simulink model "ExperimentTwoBD"  (R2015a)
settings: Solver=ode45  StartTime=0.0  StopTime=40.0  RelTol=1e-3
settings Model: Creator=Abdullah  LastModifiedBy=Abdullah

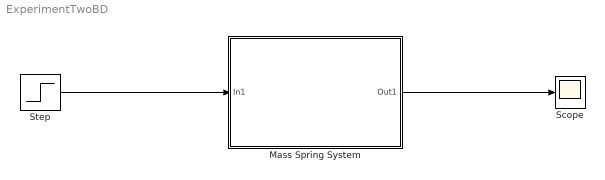
== system ExperimentTwoBD ==
  Mass Spring System : Subsystem
  Scope : Scope
  Step : Step  Time=0  SampleTime=0.01
  wires:
  Step/1 -> Mass Spring System/1(In1)
  Mass Spring System/1(Out1) -> Scope/1

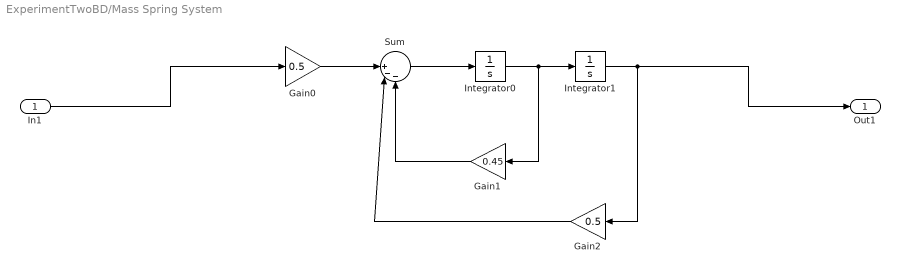
== system ExperimentTwoBD/Mass Spring System ==
  In1 : Inport
  Gain0 : Gain  Gain=0.5
  Gain1 : Gain  Gain=0.45
  Gain2 : Gain  Gain=0.5
  Integrator0 : Integrator
  Integrator1 : Integrator
  Sum : Sum  Inputs=||+--
  Out1 : Outport
  wires:
  Gain2/1 -> Sum/2
  Gain0/1 -> Sum/1
  Sum/1 -> Integrator0/1
  Integrator1/1 -> Out1/1, Gain2/1
  Gain1/1 -> Sum/3
  In1/1 -> Gain0/1
  Integrator0/1 -> Gain1/1, Integrator1/1
